simulink model "ex_codegen_dsp"  (R2020b)
settings: Solver=FixedStepDiscrete  StartTime=0.0  StopTime=60  RelTol=1e-3
libraries: dspsrcs4 x2, dspadpt3 x1, dspfdesign x1
CloseFcn:
  | clear filter_wts;
  | clear tout;
settings Model: ModifiedByFormat=The MathWorks Inc.  Creator=The MathWorks, Inc.  LastModifiedBy=The MathWorks Inc.
settings DataIOCC: LimitDataPoints=on  SaveFormat=Array  ReturnWorkspaceOutputs=off
settings OptimizationCC: ExpressionDepthLimit=2147483647  ZeroExternalMemoryAtStartup=off  ZeroInternalMemoryAtStartup=off  LifeSpan=inf
settings DebuggingCC: UnderspecifiedInitializationDetection=Classic  MergeDetectMultiDrivingBlocksExec=none  SolverPrmCheckMsg=warning  FcnCallInpInsideContextMsg=warning  StateNameClashWarn=warning  SFUnexpectedBacktrackingDiag=warning  SFNoUnconditionalDefaultTransitionDiag=warning  SFExecutionAtInitializationDiag=none  ArithmeticOperatorsInVariantConditions=warning
settings HardwareCC: ProdBitPerPointer=32  ProdBitPerSizeT=32  ProdBitPerPtrDiffT=32  ProdLargestAtomicFloat=None  ProdIntDivRoundTo=Undefined  ProdEndianess=Unspecified  ProdWordSize=32  ProdHWDeviceType=32-bit Generic
settings ModelReferenceCC: PropagateSignalLabelsOutOfModel=off
settings SFSimCC: SimUseLocalCustomCode=off  CustomCodeUndefinedFunction=UseInterfaceOnly
settings RTWCC: GenCodeOnly=on  GenerateReport=on  RTWUseLocalCustomCode=off  BuildConfiguration=Debug  LaunchReport=on  TargetLang=C++
settings CodeAppCC: StateflowObjectComments=on
settings GRTTargetCC: TargetLangStandard=C++03 (ISO)  CodeInterfacePackaging=C++ class
settings ConfigComp: CovMetricSettings=dw  CovSaveCumulativeToWorkspaceVar=on  CovSaveSingleToWorkspaceVar=on  CovExternalEMLEnable=off  CovSFcnEnable=off

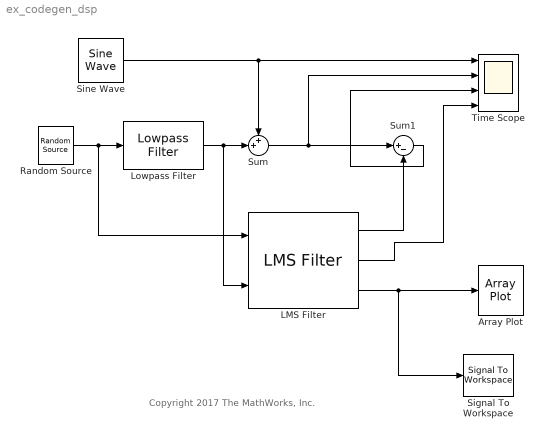
== system ex_codegen_dsp ==
  note: Copyright 2017 The MathWorks, Inc.
  Array Plot : ArrayPlot
  LMS Filter : dspadpt3/LMS Filter  Algo=Normalized LMS  L=32  stepflag=Dialog  mu=0.1  leakage=1.0  ic=0  Adapt=off  resetflag=None  weights=on  addnparflag=off  roundingMode=Floor  overflowMode=off  secondCoeffMode=Binary point scaling  secondCoeffWordLength=2  secondCoeffFracLength=15  prodOutput2Mode=Binary point scaling  prodOutput2FracLength=20  prodOutput3Mode=Binary point scaling  prodOutput3FracLength=20  prodOutput4Mode=Binary point scaling  prodOutput4FracLength=20  quotientMode=Binary point scaling  quotientFracLength=20  accum2Mode=Binary point scaling  accum2FracLength=20
      settings: SourceProductName=DSP System Toolbox
  Lowpass Filter : dspfdesign/Lowpass Filter  FilterType=FIR  DesignForMinimumOrder=on  FilterOrder=31  PassbandFrequency=8e3  StopbandFrequency=12e3  PassbandRipple=0.1  StopbandAttenuation=80  InheritSampleRate=off  SampleRate=44100  SimulateUsing=Interpreted execution  roundingMode=Floor  coeffsDataTypeStr=fixdt(1,16)
  Random Source : dspsrcs4/Random Source  SrcType=Gaussian  NormMethod=Ziggurat  CltLength=12  MinVal=0  MaxVal=1  MeanVal=0  VarVal=1  RepMode=Specify seed  rawSeed=[23341]  IsInherit=off  SampMode=Discrete  SampTime=0.05  SampFrame=1  DataType=Double  OutComplex=Real  OutputFrames=on
  Signal To Workspace : SignalToWorkspace  VariableName=filter_wts
      settings: CopyFcn=dspblkcopystw(gcbh);  Save2DSignal=3-D array (concatenate along third dimension)
  Sine Wave : dspsrcs4/Sine Wave  Amplitude=1  Frequency=0.5  Phase=0  SampleMode=Discrete  OutComplex=Real  CompMethod=Trigonometric fcn  TableSize=Speed  SampleTime=0.05  SamplesPerFrame=1  ResetState=Restart at time zero  OutputFrames=on  dataType=double  wordLen=16  udDataType=sfix(16)  fracBitsMode=Best precision  numFracBits=15  OutDataTypeStr=double  LastOutDataTypeStr=double
  Sum : Sum  Inputs=++|
  Sum1 : Sum  Inputs=|+-
  Time Scope : Scope  NumInputPorts=4
  wires:
  Sine Wave/1 -> Time Scope/1, Sum/1
  Random Source/1 -> LMS Filter/1, Lowpass Filter/1
  Sum/1 -> Time Scope/2, Sum1/1
  Lowpass Filter/1 -> LMS Filter/2, Sum/2
  LMS Filter/1 -> Sum1/2
  Sum1/1 -> Time Scope/3
  LMS Filter/2 -> Time Scope/4
  LMS Filter/3 -> Array Plot/1, Signal To Workspace/1
